simulink model "DOO_Mode_Working_might_be_mistakes"  (R2020a)
settings: Solver=FixedStepAuto  StartTime=0.0  StopTime=10.0  FixedStep=1e-3  RelTol=1e-3  EnableMultiTasking=on
undefined symbols (not defined in the file): D0, D1, D10, D11, D12, D13, D2, D3, D4, D5, D6, D7, D8, D9, PTA0, PTA1, PTA2, PTB23, PTB9, PTC16, PTC17, PTC2, PTC3, PTC4, PTD0, PTD1, PTD2, PTD3
libraries: frdmk64flib x18
settings Model: ExtModeTrigDuration=5  Creator=forre  LastModifiedBy=jeffl
settings OptimizationCC: EnhancedBackFolding=on  PassReuseOutputArgsAs=Individual arguments  ZeroExternalMemoryAtStartup=off  ZeroInternalMemoryAtStartup=off  MaxStackSize=64  OptimizeBlockOrder=speed  DifferentSizesBufferReuse=on  OptimizationCustomize=off  EfficientTunableParamExpr=on
settings DebuggingCC: ParameterTunabilityLossMsg=error
settings HardwareCC: ProdBitPerPointer=32  ProdBitPerSizeT=32  ProdBitPerPtrDiffT=32  ProdLargestAtomicInteger=Long  ProdLargestAtomicFloat=Double  ProdWordSize=32  ProdHWDeviceType=ARM Compatible->ARM Cortex
settings SFSimCC: MATLABDynamicMemAlloc=off
settings RTWCC: SystemTargetFile=ert.tlc  HardwareBoard=NXP FRDM-K64F  TemplateMakefile=ert_default_tmf  Toolchain=GNU Tools for ARM Embedded Processors
settings CodeAppCC: ForceParamTrailComments=on  IgnoreCustomStorageClasses=off  OperatorAnnotations=on  SimulinkDataObjDesc=on  SFDataObjDesc=on  InsertBlockDesc=on

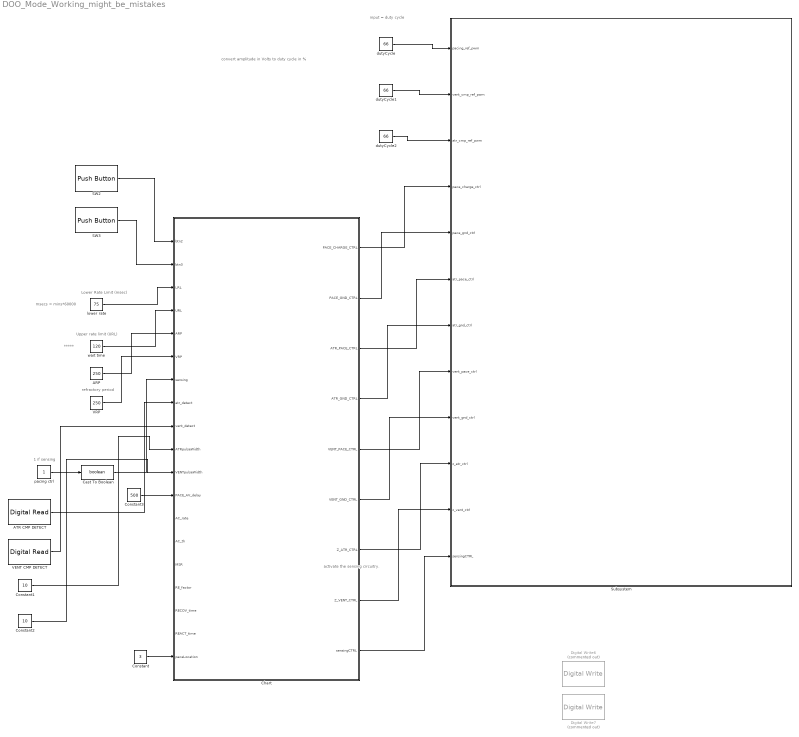
== system DOO_Mode_Working_might_be_mistakes ==
  note: convert amplitude in Volts to duty cycle in %
  note: *****
  note: msecs = mins*60000
  note: Upper rate limit (URL)
  note: refractory period
  note: Lower Rate Limit (msec)
  note: activate the sensing circuitry.
  note: input = duty cycle
  note: 1 if sensing
  ARP : Constant  Value=250
  ATR CMP DETECT : frdmk64flib/Digital Read  Whichpin=PTC16 (D0)  SampleTime=-1
  Cast To Boolean : DataTypeConversion  OutDataTypeStr=boolean
  Chart : Stateflow chart  TreatAsAtomicUnit=on
  Constant : Constant  Value=3  OutDataTypeStr=double
  Constant1 : Constant  Value=10
  Constant2 : Constant  Value=10
  Constant3 : Constant  Value=500
  Digital Write6 : frdmk64flib/Digital Write  Commented=on  Whichpin=RED_LED
  Digital Write7 : frdmk64flib/Digital Write  Commented=on  Whichpin=BLUE_LED
  SW2 : frdmk64flib/Push Button  Whichswitch=SW2  SampleTime1=-1
  SW3 : frdmk64flib/Push Button  Whichswitch=SW3  SampleTime1=-1
  Subsystem : Subsystem
  VENT CMP DETECT : frdmk64flib/Digital Read  Whichpin=PTC17 (D1)  SampleTime=-1
  VRP : Constant  Value=250
  dutyCycle : Constant  Value=66
  dutyCycle1 : Constant  Value=66
  dutyCycle2 : Constant  Value=66
  lower rate : Constant  Value=75
  pacing ctrl : Constant
  wait time : Constant  Value=120
  wires:
  dutyCycle/1 -> Subsystem/1(pacing_ref_pwm)
  SW2/1 -> Chart/1(btn2)
  Chart/4(ATR_GND_CTRL) -> Subsystem/7(atr_gnd_ctrl)
  Constant1/1 -> Chart/10(ATRpulseWidth)
  Chart/3(ATR_PACE_CTRL) -> Subsystem/6(atr_pace_ctrl)
  Chart/1(PACE_CHARGE_CTRL) -> Subsystem/4(pace_charge_ctrl)
  Chart/2(PACE_GND_CTRL) -> Subsystem/5(pace_gnd_ctrl)
  lower rate/1 -> Chart/3(LRL)
  Chart/5(VENT_PACE_CTRL) -> Subsystem/8(vent_pace_ctrl)
  Chart/6(VENT_GND_CTRL) -> Subsystem/9(vent_gnd_ctrl)
  Chart/7(Z_ATR_CTRL) -> Subsystem/10(z_atr_ctrl)
  Chart/8(Z_VENT_CTRL) -> Subsystem/11(" z_vent_ctrl")
  pacing ctrl/1 -> Cast To Boolean/1
  ATR CMP DETECT/1 -> Chart/8(atr_detect)
  VENT CMP DETECT/1 -> Chart/9(vent_detect)
  dutyCycle1/1 -> Subsystem/2(vent_cmp_ref_pwm)
  dutyCycle2/1 -> Subsystem/3(atr_cmp_ref_pwm)
  Chart/9(sensingCTRL) -> Subsystem/12(sensingCTRL)
  Cast To Boolean/1 -> Chart/7(sensing)
  ? -> Digital Write6/1
  ? -> Digital Write7/1
  SW3/1 -> Chart/2(btn3)
  wait time/1 -> Chart/4(URL)
  ARP/1 -> Chart/5(ARP)
  VRP/1 -> Chart/6(VRP)
  Constant2/1 -> Chart/11(VENTpulseWidth)
  Constant/1 -> Chart/19(paceLocation)
  Constant3/1 -> Chart/12(PACE_AV_delay)

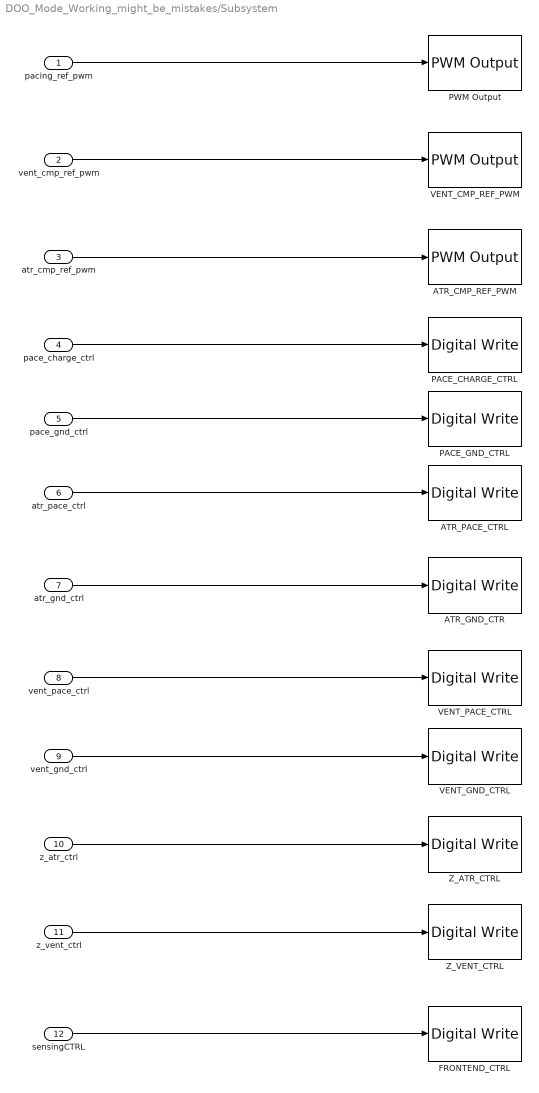
== system DOO_Mode_Working_might_be_mistakes/Subsystem ==
  pacing_ref_pwm : Inport
  vent_cmp_ref_pwm : Inport  Port=2
  atr_cmp_ref_pwm : Inport  Port=3
  pace_charge_ctrl : Inport  Port=4
  pace_gnd_ctrl : Inport  Port=5
  atr_pace_ctrl : Inport  Port=6
  atr_gnd_ctrl : Inport  Port=7
  vent_pace_ctrl : Inport  Port=8
  vent_gnd_ctrl : Inport  Port=9
  z_atr_ctrl : Inport  Port=10
  " z_vent_ctrl" : Inport  Port=11
  sensingCTRL : Inport  Port=12
  ATR_CMP_REF_PWM : frdmk64flib/PWM Output  Whichpin=PTC2 (D6)  InitialFrequency=2000  InitialDutyCycle=50
  ATR_GND_CTR : frdmk64flib/Digital Write  Whichpin=PTD2 (D11)
  ATR_PACE_CTRL : frdmk64flib/Digital Write  Whichpin=PTA0 (D8)
  FRONTEND_CTRL : frdmk64flib/Digital Write  Whichpin=PTD1 (D13)
  PACE_CHARGE_CTRL : frdmk64flib/Digital Write  Whichpin=PTB9 (D2)
  PACE_GND_CTRL : frdmk64flib/Digital Write  Whichpin=PTD0 (D10)
  PWM Output : frdmk64flib/PWM Output  Whichpin=PTA2 (D5)  InitialFrequency=2000  InitialDutyCycle=50
  VENT_CMP_REF_PWM : frdmk64flib/PWM Output  Whichpin=PTA1 (D3)  InitialFrequency=2000  InitialDutyCycle=50
  VENT_GND_CTRL : frdmk64flib/Digital Write  Whichpin=PTD3 (D12)
  VENT_PACE_CTRL : frdmk64flib/Digital Write  Whichpin=PTC4 (D9)
  Z_ATR_CTRL : frdmk64flib/Digital Write  Whichpin=PTB23 (D4)
  Z_VENT_CTRL : frdmk64flib/Digital Write  Whichpin=PTC3 (D7)
  wires:
  pace_gnd_ctrl/1 -> PACE_GND_CTRL/1
  atr_pace_ctrl/1 -> ATR_PACE_CTRL/1
  pace_charge_ctrl/1 -> PACE_CHARGE_CTRL/1
  atr_gnd_ctrl/1 -> ATR_GND_CTR/1
  vent_pace_ctrl/1 -> VENT_PACE_CTRL/1
  vent_gnd_ctrl/1 -> VENT_GND_CTRL/1
  z_atr_ctrl/1 -> Z_ATR_CTRL/1
  " z_vent_ctrl"/1 -> Z_VENT_CTRL/1
  sensingCTRL/1 -> FRONTEND_CTRL/1
  pacing_ref_pwm/1 -> PWM Output/1
  vent_cmp_ref_pwm/1 -> VENT_CMP_REF_PWM/1
  atr_cmp_ref_pwm/1 -> ATR_CMP_REF_PWM/1

== stateflow chart DOO_Mode_Working_might_be_mistakes/Chart ==
  note: beat sensed
  state SENSING_VENT_TRUE
    entry:
    sensingCTRL = true;
  state VENT_CHARGING_AND_DISCHARGE
    entry:
    % for this state paceLocation = 1
    %begin charge and discharge cycle for ventricle
    msecPerPace = 60000/RE; %new value in msec
    sensingCTRL = sensing; %enables the sensing circuitry if sensing = 1. Controled by input "sensing"
    ATR_PACE_CTRL = false;
    VENT_PACE_CTRL = false;
    PACE_CHARGE_CTRL = true;
    PACE_GND_CTRL = true;
    Z_VENT_CTRL = false;
    Z_ATR_CTRL = false
    VENT_GND_CTRL = true;
    ATR_GND_CTRL = false;
  state VENT_PACING
    entry:
    % pace ventricle
    PACE_GND_CTRL = true;
    VENT_PACE_CTRL = true;
    VENT_GND_CTRL = false;
    Z_VENT_CTRL = false;
    Z_ATR_CTRL = false;
    ATR_GND_CTRL = false;
    ATR_PACE_CTRL = false;
    sensingCTRL = sensing; %enables the sensing circuitry if sensing = 1. Controled by input "sensing"
  note: VENT PACING
  state RECOVERY_V
    RE = RE - RE_factor
    % RE factor need to time a rate (unit ppm)
    %it is depend on LRL and MSR values
  state REACTION_V
    RE = RE + RE_factor;
    % RE factor need to time a rate (unit ppm)
    %it is depend on LRL and MSR values
  note: SWITCH TO AOO, AAI,AOOR,AAIR
  note: SWITCH TO VOO,VVI,VOOR,VVIR
  state ATR_PACING
    entry:
    % pace atrium
    PACE_GND_CTRL = true;
    VENT_PACE_CTRL = false;
    VENT_GND_CTRL = false;
    Z_VENT_CTRL = false;
    Z_ATR_CTRL = false;
    ATR_GND_CTRL = false;
    ATR_PACE_CTRL = true;
    sensingCTRL = sensing; %enables the sensing circuitry if sensing = 1. Controled by input "sensing"
  state ATR_CHARGING_AND_DISCHARGE
    entry:
    % for this state paceLocation = 0
    %begin charge and discharge cycle for atrium
    msecPerPace = 60000/RE; %new value for pace timing with msec units
    sensingCTRL = sensing; %enables the sensing circuitry if sensing = 1. Controled by input "sensing"
    ATR_PACE_CTRL = false;
    VENT_PACE_CTRL = false;
    PACE_CHARGE_CTRL = true;
    PACE_GND_CTRL = true;
    Z_VENT_CTRL = false;
    Z_ATR_CTRL = false;
    VENT_GND_CTRL = false;
    ATR_GND_CTRL = true;
  note: ATR PACING
  note: SWITCH TO DOO,DOOR
  note: SWITCH TO VOO,VVI,VOOR,VVIR
  state RECOVERY_A
    RE = RE - RE_factor
    % RE factor need to time a rate (unit ppm)
    %it is depend on LRL and MSR values
  note: beat sensed
  state SENSING_ATR_TRUE
    entry:
    sensingCTRL = true;
  state REACTION_A
    RE = RE + RE_factor;
    % RE factor need to time a rate (unit ppm)
    %it is depend on LRL and MSR values
  note: SWITCH TO DOO,DOOR
  note: SWITCH TO AOO, AAI,AOOR,AAIR
  state DUAL_ATR_CHARGING_AND_DISCHARGE
    entry:
    msecPerPace = 60000/RE;
    % for this state paceLocation = 3
    %begin charge and discharge cycle for atrium
    ATR_PACE_CTRL = false;
    VENT_PACE_CTRL = false;
    PACE_CHARGE_CTRL = true;
    PACE_GND_CTRL = true;
    Z_VENT_CTRL = false;
    Z_ATR_CTRL = false;
    VENT_GND_CTRL = false;
    ATR_GND_CTRL = true;
  state DUAL_ATR_PACING
    entry:
    % pace atrium
    PACE_GND_CTRL = true;
    VENT_PACE_CTRL = false;
    VENT_GND_CTRL = false;
    Z_VENT_CTRL = false;
    Z_ATR_CTRL = false;
    ATR_GND_CTRL = false;
    ATR_PACE_CTRL = true;
    AP_flag = true; % rise to true when Atrium have a pace
  note: DOO,DOOR
  state DUAL_VENT_PACING
    entry:
    % pace ventricle
    PACE_GND_CTRL = true;
    VENT_PACE_CTRL = true;
    VENT_GND_CTRL = false;
    Z_VENT_CTRL = false;
    Z_ATR_CTRL = false;
    ATR_GND_CTRL = false;
    ATR_PACE_CTRL = false;
    sensingCTRL = sensing; %enables the sensing circuitry if sensing = 1. Controled by input "sensing"
    AP_flag = false;
  state DUAL_VENT_CHARGING_AND_DISCHARGE
    entry:
    %begin charge and discharge cycle for ventricle
    msecPerPace = 60000/RE; %new value in msec
    sensingCTRL = sensing; %enables the sensing circuitry if sensing = 1. Controled by input "sensing"
    ATR_PACE_CTRL = false;
    VENT_PACE_CTRL = false;
    PACE_CHARGE_CTRL = true;
    PACE_GND_CTRL = true;
    Z_VENT_CTRL = false;
    Z_ATR_CTRL = false
    VENT_GND_CTRL = true;
    ATR_GND_CTRL = false;
  state RECOVERY_D
    RE = RE - RE_factor
    % RE factor need to time a rate (unit ppm)
    %it is depend on LRL and MSR values
  state REACTION_D
    RE = RE + RE_factor;
    % RE factor need to time a rate (unit ppm)
    %it is depend on LRL and MSR values
  VENT_CHARGING_AND_DISCHARGE -> SENSING_VENT_TRUE [order 1] : after((VRP-VENTpulseWidth),msec)[sensing && (vent_detect || btn3)]
  SENSING_VENT_TRUE -> VENT_CHARGING_AND_DISCHARGE : after(VENTpulseWidth, msec)
  VENT_CHARGING_AND_DISCHARGE -> DUAL_ATR_CHARGING_AND_DISCHARGE [order 6] : [(paceLocation == 3) || (paceLocation == 6)]{RE=LRL}
  VENT_PACING -> VENT_CHARGING_AND_DISCHARGE : after(VENTpulseWidth, msec)
  VENT_CHARGING_AND_DISCHARGE -> VENT_PACING [order 4] : after((msecPerPace-VENTpulseWidth), msec){PACE_CHARGE_CTRL = false;}
  VENT_CHARGING_AND_DISCHARGE -> ATR_CHARGING_AND_DISCHARGE [order 5] : [(paceLocation == 1)|| (paceLocation == 5)]{RE=LRL}
  DUAL_ATR_CHARGING_AND_DISCHARGE -> VENT_CHARGING_AND_DISCHARGE [order 6] : [(paceLocation == 2) || (paceLocation == 4)]{RE=LRL}
  RECOVERY_V -> VENT_CHARGING_AND_DISCHARGE : after(((RECOV_time/RE_factor)*60),sec)
  ATR_CHARGING_AND_DISCHARGE -> VENT_CHARGING_AND_DISCHARGE [order 6] : [(paceLocation == 2)|| (paceLocation == 4)]{RE=LRL}
  VENT_CHARGING_AND_DISCHARGE -> RECOVERY_V [order 3] : [[AC_rate>AC_th&&LRL>MSR]&&(paceLocation==4)]
  VENT_CHARGING_AND_DISCHARGE -> REACTION_V [order 2] : [(AC_rate<AC_th)&&LRL<MSR&&(paceLocation==4)]
  REACTION_V -> VENT_CHARGING_AND_DISCHARGE : after((REACT_time/RE_factor),sec)
  (default) -> ATR_CHARGING_AND_DISCHARGE : {RE = LRL}
  ATR_CHARGING_AND_DISCHARGE -> (junction 282) [order 1] : [(paceLocation == 3) || (paceLocation == 6)]{RE=LRL}
  ATR_CHARGING_AND_DISCHARGE -> ATR_PACING [order 5] : after((msecPerPace-ATRpulseWidth), msec){PACE_CHARGE_CTRL = false;}
  ATR_PACING -> ATR_CHARGING_AND_DISCHARGE : after(ATRpulseWidth, msec)
  RECOVERY_A -> ATR_CHARGING_AND_DISCHARGE : after(((RECOV_time/RE_factor)*60),sec)
  ATR_CHARGING_AND_DISCHARGE -> RECOVERY_A [order 4] : [[AC_rate>AC_th&&LRL>MSR]&&(paceLocation==5)]
  REACTION_A -> ATR_CHARGING_AND_DISCHARGE : after((REACT_time/RE_factor),sec)
  ATR_CHARGING_AND_DISCHARGE -> SENSING_ATR_TRUE [order 2] : after((ARP-ATRpulseWidth),msec)[sensing && (atr_detect || btn3)]
  SENSING_ATR_TRUE -> ATR_CHARGING_AND_DISCHARGE : after(ATRpulseWidth, msec)
  DUAL_ATR_CHARGING_AND_DISCHARGE -> ATR_CHARGING_AND_DISCHARGE [order 5] : [(paceLocation == 1)|| (paceLocation == 5)]{RE=LRL}
  ATR_CHARGING_AND_DISCHARGE -> REACTION_A [order 3] : [(AC_rate<AC_th)&&LRL<MSR&&(paceLocation==5)]
  (junction 282) -> DUAL_ATR_CHARGING_AND_DISCHARGE : {AP_flag == false}
  DUAL_ATR_CHARGING_AND_DISCHARGE -> DUAL_ATR_PACING [order 2] : [AP_flag == false]{PACE_CHARGE_CTRL = false;}
  DUAL_ATR_PACING -> DUAL_ATR_CHARGING_AND_DISCHARGE : after( ATRpulseWidth, msec)
  DUAL_ATR_CHARGING_AND_DISCHARGE -> (junction 285) [order 1] : [AP_flag == true]
  (junction 285) -> DUAL_VENT_CHARGING_AND_DISCHARGE : after(PACE_AV_delay-ATRpulseWidth,msec)
  (junction 288) -> DUAL_ATR_CHARGING_AND_DISCHARGE : [AP_flag == false]
  DUAL_ATR_CHARGING_AND_DISCHARGE -> REACTION_D [order 3] : [(AC_rate<AC_th)&&LRL<MSR&&(paceLocation==6)]
  REACTION_D -> DUAL_ATR_CHARGING_AND_DISCHARGE : after((REACT_time/RE_factor),sec)
  DUAL_ATR_CHARGING_AND_DISCHARGE -> RECOVERY_D [order 4] : [(AC_rate>AC_th)&&(LRL>MSR)&&(paceLocation==6)]
  RECOVERY_D -> DUAL_ATR_CHARGING_AND_DISCHARGE : after(((RECOV_time/RE_factor)*60),sec)
  DUAL_VENT_PACING -> DUAL_VENT_CHARGING_AND_DISCHARGE : after((VENTpulseWidth), msec)
  DUAL_VENT_CHARGING_AND_DISCHARGE -> DUAL_VENT_PACING [order 1] : [AP_flag == true]{PACE_CHARGE_CTRL = false;}
  DUAL_VENT_CHARGING_AND_DISCHARGE -> (junction 288) [order 2] : after(msecPerPace-VENTpulseWidth-PACE_AV_delay,msec)
  data: PACE_CHARGE_CTRL output boolean; PACE_GND_CTRL output boolean; btn2 input boolean; btn3 input boolean; ATR_PACE_CTRL output boolean; ATR_GND_CTRL output boolean; LRL input double; URL input double; ARP input double; VRP input double; VENT_PACE_CTRL output boolean; VENT_GND_CTRL output boolean; Z_ATR_CTRL output boolean; Z_VENT_CTRL output boolean; sensing input boolean; atr_detect input boolean; vent_detect input boolean; sensingCTRL output boolean; msecPerPace local double; ATRpulseWidth input double; VENTpulseWidth input double; PACE_AV_delay input double; AP_flag local boolean; AC_rate input double; AC_th input double; MSR input double; RE_factor input double; RECOV_time input double; REACT_time input double; RE local double; paceLocation input double
  data atr_detect settings: description=|
      | 0 = pace atrium
      | 1 = pace ventricle
  data vent_detect settings: description=|
      | 0 = pace atrium
      | 1 = pace ventricle
  data paceLocation settings: description=|
      | 0 = pace atrium
      | 1 = pace ventricle
